simulink model "contrilled_rectifier_zcd"  (R2025a)
settings: Solver=ode4  StartTime=0.0  StopTime=1  FixedStep=1e-6  RelTol=1e-3
libraries: spsThyristorLib x4, spsVoltageMeasurementLib x2, spsACVoltageSourceLib x1, spsBreakerLib x1, spsSeriesRLCBranchLib x1, simulink x1, sps_lib x1
settings Model: Creator=ketan  LastModifiedBy=ketan

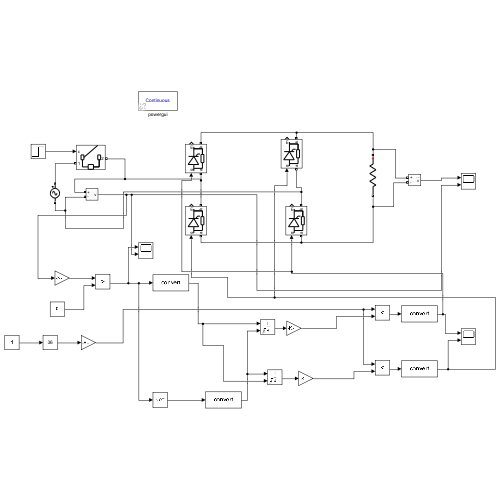
[thumbnail: Simulink's stored preview of the top-level diagram]
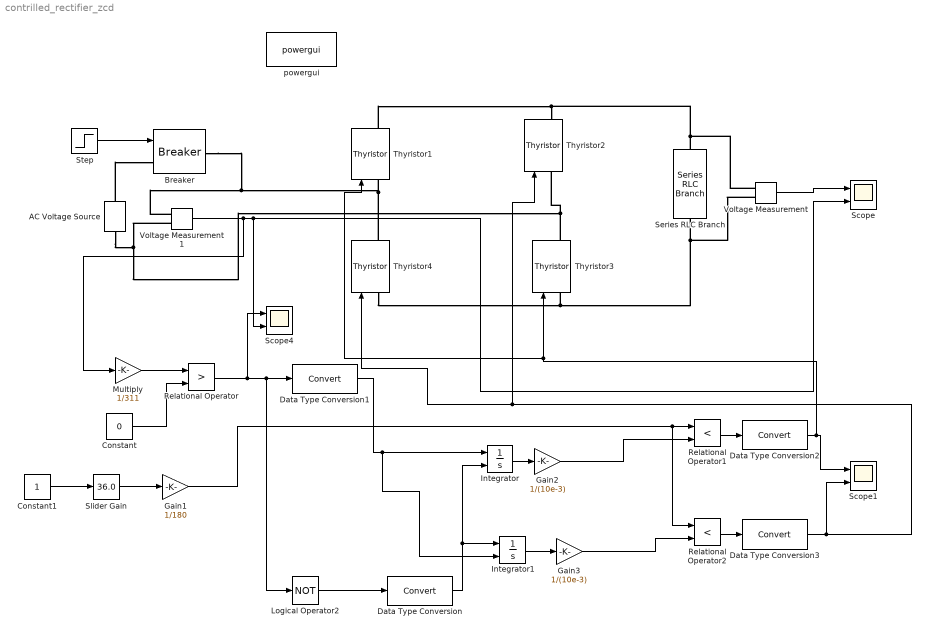
== system contrilled_rectifier_zcd ==
  AC Voltage Source : spsACVoltageSourceLib/AC Voltage Source  Amplitude=311  Phase=0  Frequency=50  SampleTime=0  Measurements=None  BusType=swing  Pref=10e3  Qref=0  Qmin=-inf  Qmax=+inf
  Breaker : spsBreakerLib/Breaker  InitialState=0  SwitchingTimes="[1/60  5/60]"  External=on  BreakerResistance=0.01  SnubberResistance=1e6  SnubberCapacitance=inf  Measurements=Branch voltage  MoreParameters=on  NoBreakLoop=off
  Constant : Constant  Value=0
  Constant1 : Constant
  Data Type Conversion{,1..3} (4 alike) : DataTypeConversion  SaturateOnIntegerOverflow=off  RndMeth=Floor
  Gain1 : Gain  Gain=1/180
  Gain2 : Gain  Gain=1/(10e-3)
  Gain3 : Gain  Gain=1/(10e-3)
  Integrator : Integrator  ExternalReset=rising
  Integrator1 : Integrator  ExternalReset=rising
  Logical Operator2 : Logic  Operator=NOT  AllPortsSameDT=off  OutDataTypeStr=boolean
  Multiply : Gain  Gain=1/311
  Relational Operator : RelationalOperator  Operator=>  OutDataTypeStr=boolean  RndMeth=Ceiling  InputSameDT=off
  Relational Operator1 : RelationalOperator  Operator=<  OutDataTypeStr=boolean  RndMeth=Simplest  InputSameDT=off
  Relational Operator2 : RelationalOperator  Operator=<  OutDataTypeStr=boolean  RndMeth=Simplest  InputSameDT=off
  Scope : Scope  NumInputPorts=2
      settings: ActiveDisplayYMinimum=-34.910333812019083  ActiveDisplayYMaximum=389.75951433080394
  Scope1 : Scope  NumInputPorts=2
      settings: ActiveDisplayYMinimum=-0.15465784215784212  ActiveDisplayYMaximum=1.0953421578421578
  Scope4 : Scope  NumInputPorts=2
      settings: ActiveDisplayYMinimum=-4.5948642093673726  ActiveDisplayYMaximum=2.90799960404107  DataLoggingVariableName=ScopeData4
  Series RLC Branch : spsSeriesRLCBranchLib/Series RLC Branch  LConnTagsString=__new0  RConnTagsString=__new0  BranchType=R  Resistance=1000  Inductance=1e-3  SetiL0=off  InitialCurrent=0  Capacitance=1e-6  Setx0=off  InitialVoltage=0  Measurements=None
  Slider Gain : simulink/Math Operations/Slider Gain  gain=36.0  low=0  high=90
  Step : Step  Time=0.5  SampleTime=0
  Thyristor{1..4} (4 alike) : spsThyristorLib/Thyristor  Ron=0.001  Lon=0  Vf=0.8  IC=0  Rs=500  Cs=250e-9  Measurements=on
  Voltage Measurement : spsVoltageMeasurementLib/Voltage Measurement  PhasorSimulation=off  OutputType=Complex  PSBequivalent=0
  Voltage Measurement1 : spsVoltageMeasurementLib/Voltage Measurement  PhasorSimulation=off  OutputType=Complex  PSBequivalent=0
  powergui : sps_lib/powergui  Priority=1  SimulationMode=Continuous  SampleTime=50e-6  frequency=60  Iterations=50  frequencyindice=50  Pbase=100e6  ErrMax=1e-4  UnitsV=kV  UnitsW=MW  buscounter=0  FunctionMessages=off  echomessages=off  EnableUseOfTLC=off  CurrentSourceSwitches=off  DisableSnubberDevices=off  DisableRonSwitches=off  DisableVfSwitches=off  DisplayEquations=off  AutomaticDiscreteSolvers=off  SolverType=Tustin/Backward Euler (TBE)  Interpol=off  ExternalGateDelay=off  methode=off  Ts=100  x0status=blocks  SPID=on  SwTol=0  HookPort=off  NonlinearTolerance=1e-4  nMaxIteration=100  ContinueOnMaxIteration=off  RestoreLinks=warning  ResistiveCurrentMeasurement=off  Frange=[0:2:500]  Ylog=off  Xlog=on  ShowGrid=off  save=off  variable=ZData  structure=0  ZoomFFT=off  StartTime=0.0  cycles=1  DisplayStyle=1  fundamental=60  FreqAxis=off  MaxFrequency=1000  frequencyindicesteady=1  RmsSteady=1  display=off
  wires:
  Voltage Measurement/1 -> Scope/1
  Step/1 -> Breaker/1
  Voltage Measurement1/1 -> Multiply/1, Scope/2, Scope4/2
  Constant/1 -> Relational Operator/2
  Relational Operator/1 -> Scope4/1, Data Type Conversion1/1, Logical Operator2/1
  Logical Operator2/1 -> Data Type Conversion/1
  Constant1/1 -> Slider Gain/1
  Slider Gain/1 -> Gain1/1
  Gain1/1 -> Relational Operator2/1, Relational Operator1/1
  Integrator/1 -> Gain2/1
  Integrator1/1 -> Gain3/1
  Gain3/1 -> Relational Operator2/2
  Gain2/1 -> Relational Operator1/2
  Relational Operator1/1 -> Data Type Conversion2/1
  Relational Operator2/1 -> Data Type Conversion3/1
  Data Type Conversion/1 -> Integrator1/1, Integrator/2
  Data Type Conversion1/1 -> Integrator1/2, Integrator/1
  Data Type Conversion2/1 -> Scope1/1, Thyristor1/1, Thyristor3/1
  Data Type Conversion3/1 -> Scope1/2, Thyristor2/1, Thyristor4/1
  Multiply/1 -> Relational Operator/1
  connections:
  Thyristor1/RConn1 -- Voltage Measurement/LConn1 -- Series RLC Branch/LConn1 -- Thyristor2/RConn1
  Thyristor4/LConn1 -- Voltage Measurement/LConn2 -- Series RLC Branch/RConn1 -- Thyristor3/LConn1
  Thyristor3/RConn1 -- AC Voltage Source/LConn1 -- Voltage Measurement1/LConn2 -- Thyristor2/LConn1
  Thyristor4/RConn1 -- Breaker/RConn1 -- Voltage Measurement1/LConn1 -- Thyristor1/LConn1
  AC Voltage Source/RConn1 -- Breaker/LConn1
